simulink model "model_matematyczny_2018a"  (R2022a)
settings: Solver=VariableStepAuto  StartTime=0.0  StopTime=30  RelTol=1e-3
settings Model: Creator=Admin  LastModifiedBy=dawid
settings SolverCC: AlgebraicLoopSolver=TrustRegion
settings DebuggingCC: ArithmeticOperatorsInVariantConditions=warning
settings SFSimCC: CustomCodeUndefinedFunction=UseInterfaceOnly

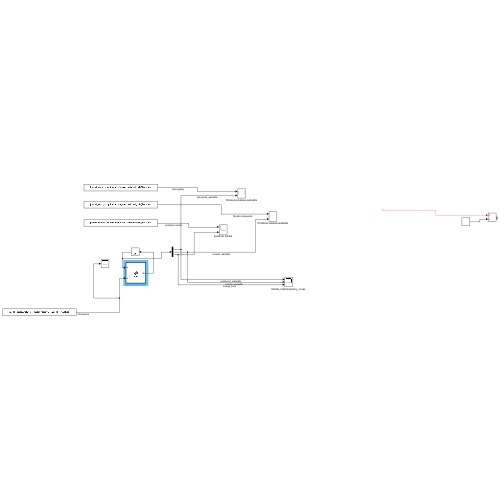
[thumbnail: Simulink's stored preview of the top-level diagram]
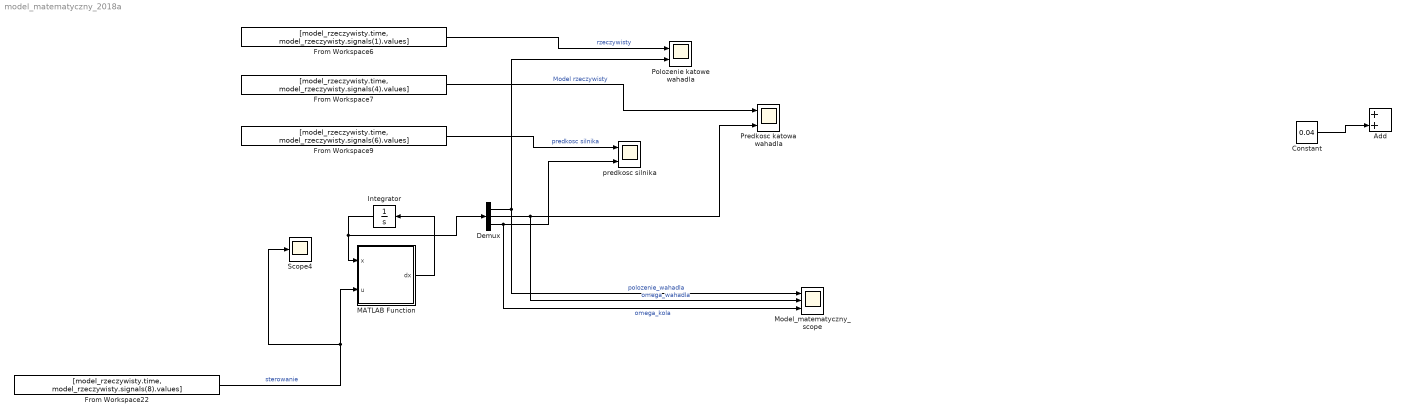
== system model_matematyczny_2018a ==
  Add : Sum
  Constant : Constant  Value=0.04
  Demux : Demux  Outputs=3
  From Workspace22 : FromWorkspace  VariableName=[model_rzeczywisty.time, model_rzeczywisty.signals(8).values]
  From Workspace6 : FromWorkspace  VariableName=[model_rzeczywisty.time, model_rzeczywisty.signals(1).values]
  From Workspace7 : FromWorkspace  VariableName=[model_rzeczywisty.time, model_rzeczywisty.signals(4).values]
  From Workspace9 : FromWorkspace  VariableName=[model_rzeczywisty.time, model_rzeczywisty.signals(6).values]
  Integrator : Integrator  InitialCondition=[0, 0, 0]
  MATLAB Function : MATLAB Function  TreatAsAtomicUnit=on
  Model_matematyczny_scope : Scope  NumInputPorts=3
  "Polozenie katowe wahadla " : Scope  NumInputPorts=2
  "Predkosc katowa wahadla " : Scope  NumInputPorts=2
  Scope4 : Scope
  "predkosc silnika " : Scope  NumInputPorts=2
  wires:
  MATLAB Function/1(dx) -> Integrator/1
  Integrator/1 -> MATLAB Function/1(x), Demux/1
  Demux/2 -> Model_matematyczny_scope/2, "Predkosc katowa wahadla "/2  "omega_wahadla"
  Demux/3 -> Model_matematyczny_scope/3, "predkosc silnika "/2  "omega_kola"
  Demux/1 -> "Polozenie katowe wahadla "/2, Model_matematyczny_scope/1  "polozenie_wahadla"
  ? -> Add/1
  Constant/1 -> Add/2
  From Workspace6/1 -> "Polozenie katowe wahadla "/1  "rzeczywisty"
  From Workspace7/1 -> "Predkosc katowa wahadla "/1  "Model rzeczywisty"
  From Workspace9/1 -> "predkosc silnika "/1  "predkosc silnika"
  From Workspace22/1 -> MATLAB Function/2(u), Scope4/1  "sterowanie"

== matlab function model_matematyczny_2018a/MATLAB Function ==
  data: x input; u input; dx output
% function dx = fcn(x, u)
% 
% %dane wyidentyfikowane
% MgL = 0.1064;
% g = 9.81;
% kt = 0.027; % NmA
% R = 0.4; %Ohmy
% 
% mi_phi = 0.000082; 
% % mi_phi = 1.566850664740816e-04;
% % mi_theta = 0.0290; %zostało wyznaczone z drgań swobodnych 
% mi_theta = 0.0290;
% 
% G = 488.7;
% J = 0.0283; %kg*m^2
% 
% %wspołczynnik a:
% % a = 0.0023;
% % b = -0.0022;
% p = [0.002321260244060,-0.002210724041962];
% dx = [0 0 0];
% dx(1) = x(2); % pochodna polozenia
% dx(2) = (1/J)*(MgL * sin(x(1)) - mi_theta * x(2) + (((kt * kt)/R) + mi_phi) * x(3) - kt*u/R); % pochodna predkosci obrotowe belki
% dx(3) = G * (u - polyval(p, x(3))); %pochodna predkosci smigla 
% 
% end


function dx = fcn(x, u)

%dane wyidentyfikowane
MgL = 0.1264;
g = 9.81;
kt = 0.027; % NmA
ke = 0.025;
R = 2.4; %Ohmy

% mi_phi = 0.000644785835713765; 
mi_phi = 0.0000882;
% mi_theta = 0.00000132; %zostało wyznaczone z drgań swobodnych 
mi_theta = 0.0290;

G = 488.648;
J = 0.0219; %kg*m^2
% J = 0.0254;
p = [0.002314296507890,-8.816367649105842e-04];
p_volt = [11.823766233766237,0.009523809523809];
dx = [0 0 0];
dx(1) = x(2); % pochodna polozenia
% dx(2) = (1/J)*(-MgL * sin(x(1)) - mi_theta * x(2) + (((kt * ke)/R) + mi_phi) * x(3) - kt*u/R); % pochodna predkosci obrotowe belki
dx(2) = (1/J)*(-MgL * sin(x(1)) - mi_theta * x(2) - (kt * (polyval(p_volt, u) - ke * x(3)) / R) + mi_phi * x(3));
dx(3) = G * (u - polyval(p, x(3))); %pochodna predkosci smigla 

end
